simulink library "earthHorizonSensorHW_sl"  (R2024b)
settings: Solver=VariableStepAuto  StartTime=0.0  StopTime=10.0  RelTol=1e-3
undefined symbols (not defined in the file): earthHorizonErrorDcm, earthHorizonErrorFlag
settings Model: Creator=gilbu
settings RTWCC: GPUComputeCapability=3.5

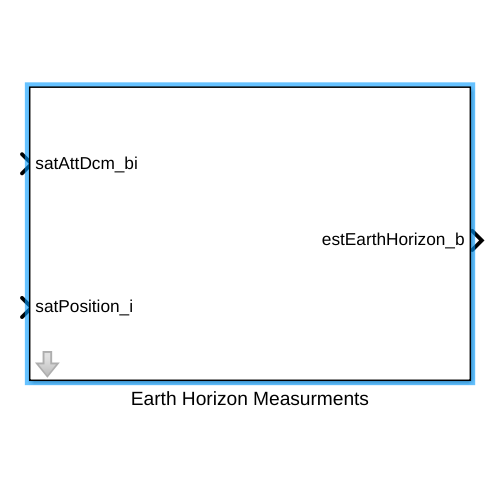
[thumbnail: Simulink's stored preview of the top-level diagram]
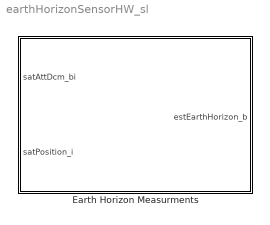
== system earthHorizonSensorHW_sl ==
  Earth Horizon Measurments : Subsystem  mask{earthHorizonErrorFlag=earthHorizonErrorFlag, earthHorizonErrorDcm=earthHorizonErrorDcm}
      mask prompts: earthHorizonErrorFlag "Earth Horizon Error Flag <1> [-]"; earthHorizonErrorDcm "Constant Measurment Error <3,3> [rad]"
      mask DialogControl DescTextVar Prompt: Simulated Earth Horizon sensor HW for attitude measurements. Error includes constant 3-axis angular error. Errors can be tured on an off using earthHorizonErrorFlag and parameters.
      mask DialogControl Control2 Prompt: Earth Horizon Error Flag equal to one will allow guassian white noise into the attitude measurements

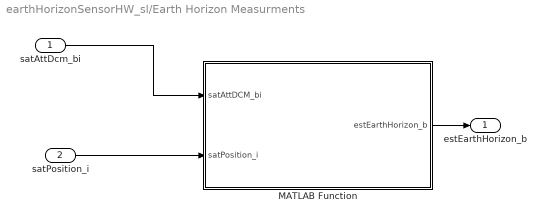
== system earthHorizonSensorHW_sl/Earth Horizon Measurments ==
  satAttDcm_bi : Inport
  satPosition_i : Inport  Port=2
  MATLAB Function : MATLAB Function  TreatAsAtomicUnit=on
  estEarthHorizon_b : Outport
  wires:
  satAttDcm_bi/1 -> MATLAB Function/1(satAttDCM_bi)
  MATLAB Function/1(estEarthHorizon_b) -> estEarthHorizon_b/1
  satPosition_i/1 -> MATLAB Function/2(satPosition_i)

== matlab function earthHorizonSensorHW_sl/Earth Horizon Measurments/MATLAB Function ==
  data: satAttDCM_bi input double size=3,3; estEarthHorizon_b output size=3; satPosition_i input size=3; earthHorizonErrorFlag parameter size=1; earthHorizonErrorDcm parameter size=3,3
% Author: Antonio Gil Buitrago
function estEarthHorizon_b = earthHorizonMeasurement( ...
    satAttDCM_bi,satPosition_i,... %inputs
   earthHorizonErrorFlag,earthHorizonErrorDcm ... % Parameters
   )

%-------------------------------------------------------------------------------
% Initialize values

% Position unit vector
unitSatPos = satPosition_i./norm(satPosition_i);



%-------------------------------------------------------------------------------
% Simulated Noise Measurement

if earthHorizonErrorFlag

   estEarthHorizon_b = earthHorizonErrorDcm*satAttDCM_bi*unitSatPos;
else
    estEarthHorizon_b = satAttDCM_bi*unitSatPos;
end

%-------------------------------------------------------------------------------
end
